simulink library "halin"  (R2021b)
settings: Solver=VariableStepAuto  StartTime=0.0  StopTime=10.0  RelTol=1e-3
undefined symbols (not defined in the file): KHAL_CAN1ABM1E2E_flg, KHAL_CAN1ESC1E2E_flg, KHAL_CAN1ESC5E2E_flg, KHAL_CAN1ESC7E2E_flg, KHAL_CAN1FCM2E2E_flg, KHAL_CAN1FCM3E2E_flg, KHAL_CAN1FCM4E2E_flg, KHAL_CAN3BMS1E2E_flg, KHAL_CAN3BMS6E2E_flg, KHAL_CAN3CCU1E2E_flg, KHAL_CAN3CCU2E2E_flg, KHAL_CAN3MCUF1E2E_flg, KHAL_CAN3MCUR1E2E_flg, KHAL_CAN3Shifter1E2E_flg, TRUE
libraries: simulink x420, FVT_lib x149, hcu_lib x49
(part 12 of 14)

== system halin/HAL_IN/CAN1/ABM1/LifeCountABM1 ==
  LifeCount_ABM1 : Inport
  UnitConverter : DataTypeConversion  OutDataTypeStr=uint8
  VHAL_LifeCountABM1_enum : Outport
  wires:
  UnitConverter/1 -> VHAL_LifeCountABM1_enum/1
  LifeCount_ABM1/1 -> UnitConverter/1

== system halin/HAL_IN/CAN1/ABM1/PsngrSeatBeltCmd ==
  PsngrSeatBeltCmd : Inport
  UnitConverter : DataTypeConversion  OutDataTypeStr=uint8
  VHAL_PsngrSeatBeltCmd_flg : Outport
  wires:
  UnitConverter/1 -> VHAL_PsngrSeatBeltCmd_flg/1
  PsngrSeatBeltCmd/1 -> UnitConverter/1

== system halin/HAL_IN/CAN1/ABM1/RCenterSeatBeltCmd ==
  RCenterSeatBeltCmd : Inport
  UnitConverter : DataTypeConversion  OutDataTypeStr=uint8
  VHAL_RCenterSeatBeltCmd_flg : Outport
  wires:
  UnitConverter/1 -> VHAL_RCenterSeatBeltCmd_flg/1
  RCenterSeatBeltCmd/1 -> UnitConverter/1

== system halin/HAL_IN/CAN1/ABM1/RDriverSeatBeltCmd ==
  RDriverSeatBeltCmd : Inport
  UnitConverter : DataTypeConversion  OutDataTypeStr=uint8
  VHAL_RDriverSeatBeltCmd_flg : Outport
  wires:
  UnitConverter/1 -> VHAL_RDriverSeatBeltCmd_flg/1
  RDriverSeatBeltCmd/1 -> UnitConverter/1

== system halin/HAL_IN/CAN1/ABM1/RPsngrSeatBeltCmd ==
  RPsngrSeatBeltCmd : Inport
  UnitConverter : DataTypeConversion  OutDataTypeStr=uint8
  VHAL_RPsngrSeatBeltCmd_flg : Outport
  wires:
  UnitConverter/1 -> VHAL_RPsngrSeatBeltCmd_flg/1
  RPsngrSeatBeltCmd/1 -> UnitConverter/1

== system halin/HAL_IN/CAN1/EPAS1/DriIntend ==
  DriIntend : Inport
  UnitConverter : DataTypeConversion  OutDataTypeStr=uint8
  VHAL_DriIntend_enum : Outport
  wires:
  UnitConverter/1 -> VHAL_DriIntend_enum/1
  DriIntend/1 -> UnitConverter/1

== system halin/HAL_IN/CAN1/EPAS1/EPSAOIControl ==
  EPS_AOI_Control : Inport
  UnitConverter : DataTypeConversion  OutDataTypeStr=uint8
  VHAL_EPSAOIControl_enum : Outport
  wires:
  UnitConverter/1 -> VHAL_EPSAOIControl_enum/1
  EPS_AOI_Control/1 -> UnitConverter/1

== system halin/HAL_IN/CAN1/EPAS2/SASAngle ==
  SAS_Angle : Inport
  UnitConverter : DataTypeConversion  OutDataTypeStr=uint16
  convert_in : FVT_lib/hal/convert_in  gain=0.1  offset=-900
  VHAL_SASAngle_Deg : Outport
  wires:
  convert_in/1 -> VHAL_SASAngle_Deg/1
  UnitConverter/1 -> convert_in/1
  SAS_Angle/1 -> UnitConverter/1

== system halin/HAL_IN/CAN1/EPAS2/SASCAL ==
  SAS_CAL : Inport
  UnitConverter : DataTypeConversion  OutDataTypeStr=uint8
  VHAL_SASCAL_flg : Outport
  wires:
  UnitConverter/1 -> VHAL_SASCAL_flg/1
  SAS_CAL/1 -> UnitConverter/1

== system halin/HAL_IN/CAN1/EPAS2/SASSpeed ==
  SAS_Speed : Inport
  UnitConverter : DataTypeConversion  OutDataTypeStr=uint8
  convert_in : FVT_lib/hal/convert_in  gain=4  offset=0
  VHAL_SASSpeed_degps : Outport
  wires:
  convert_in/1 -> VHAL_SASSpeed_degps/1
  UnitConverter/1 -> convert_in/1
  SAS_Speed/1 -> UnitConverter/1

== system halin/HAL_IN/CAN1/EPAS2/SASSpeedValid ==
  SAS_Speed_Valid : Inport
  UnitConverter : DataTypeConversion  OutDataTypeStr=uint8
  VHAL_SASSpeedValid_flg : Outport
  wires:
  UnitConverter/1 -> VHAL_SASSpeedValid_flg/1
  SAS_Speed_Valid/1 -> UnitConverter/1

== system halin/HAL_IN/CAN1/EPAS2/SASV ==
  SAS_V : Inport
  UnitConverter : DataTypeConversion  OutDataTypeStr=uint8
  VHAL_SASV_flg : Outport
  wires:
  UnitConverter/1 -> VHAL_SASV_flg/1
  SAS_V/1 -> UnitConverter/1

== system halin/HAL_IN/CAN1/EPB1/DOASta ==
  DOA_Sta : Inport
  UnitConverter : DataTypeConversion  OutDataTypeStr=uint8
  VHAL_DOASta_flg : Outport
  wires:
  UnitConverter/1 -> VHAL_DOASta_flg/1
  DOA_Sta/1 -> UnitConverter/1

== system halin/HAL_IN/CAN1/EPB1/EPBCarWashMode ==
  EPBCarWashMode : Inport
  UnitConverter : DataTypeConversion  OutDataTypeStr=uint8
  VHAL_EPBCarWashMode_flg : Outport
  wires:
  UnitConverter/1 -> VHAL_EPBCarWashMode_flg/1
  EPBCarWashMode/1 -> UnitConverter/1

== system halin/HAL_IN/CAN1/EPB1/EPBErrSta ==
  EPBErrSta : Inport
  UnitConverter : DataTypeConversion  OutDataTypeStr=uint8
  VHAL_EPBErrSta_enum : Outport
  wires:
  UnitConverter/1 -> VHAL_EPBErrSta_enum/1
  EPBErrSta/1 -> UnitConverter/1

== system halin/HAL_IN/CAN1/EPB1/EPBExtApplyAvail ==
  EPBExtApplyAvail : Inport
  UnitConverter : DataTypeConversion  OutDataTypeStr=uint8
  VHAL_EPBExtApplyAvail_flg : Outport
  wires:
  UnitConverter/1 -> VHAL_EPBExtApplyAvail_flg/1
  EPBExtApplyAvail/1 -> UnitConverter/1

== system halin/HAL_IN/CAN1/EPB1/EPBExtReleaseAvail ==
  EPBExtReleaseAvail : Inport
  UnitConverter : DataTypeConversion  OutDataTypeStr=uint8
  VHAL_EPBExtReleaseAvail_flg : Outport
  wires:
  UnitConverter/1 -> VHAL_EPBExtReleaseAvail_flg/1
  EPBExtReleaseAvail/1 -> UnitConverter/1

== system halin/HAL_IN/CAN1/EPB1/EPBSta ==
  EPBSta : Inport
  UnitConverter : DataTypeConversion  OutDataTypeStr=uint8
  VHAL_EPBSta_enum : Outport
  wires:
  UnitConverter/1 -> VHAL_EPBSta_enum/1
  EPBSta/1 -> UnitConverter/1

== system halin/HAL_IN/CAN1/ESC1/ESC1CS ==
  ESC1_CS : Inport
  UnitConverter : DataTypeConversion  OutDataTypeStr=uint8
  VHAL_ESC1CS_enum : Outport
  wires:
  UnitConverter/1 -> VHAL_ESC1CS_enum/1
  ESC1_CS/1 -> UnitConverter/1

== system halin/HAL_IN/CAN1/ESC1/ESC1RC ==
  ESC1_RC : Inport
  UnitConverter : DataTypeConversion  OutDataTypeStr=uint8
  VHAL_ESC1RC_enum : Outport
  wires:
  UnitConverter/1 -> VHAL_ESC1RC_enum/1
  ESC1_RC/1 -> UnitConverter/1

== system halin/HAL_IN/CAN1/ESC1/FrPTCSActive ==
  Fr_PTCS_Active : Inport
  UnitConverter : DataTypeConversion  OutDataTypeStr=uint8
  VHAL_FrPTCSActive_flg : Outport
  wires:
  UnitConverter/1 -> VHAL_FrPTCSActive_flg/1
  Fr_PTCS_Active/1 -> UnitConverter/1

== system halin/HAL_IN/CAN1/ESC1/FrntAxlTrqReqDrv ==
  FrntAxlTrqReq_Drv : Inport
  UnitConverter : DataTypeConversion  OutDataTypeStr=uint16
  convert_in : FVT_lib/hal/convert_in  gain=0.5  offset=-5300
  VHAL_FrntAxlTrqReqDrv_Nm : Outport
  wires:
  convert_in/1 -> VHAL_FrntAxlTrqReqDrv_Nm/1
  UnitConverter/1 -> convert_in/1
  FrntAxlTrqReq_Drv/1 -> UnitConverter/1

== system halin/HAL_IN/CAN1/ESC1/RearAxlTrqReqDrv ==
  RearAxlTrqReq_Drv : Inport
  UnitConverter : DataTypeConversion  OutDataTypeStr=uint16
  convert_in : FVT_lib/hal/convert_in  gain=0.5  offset=-5300
  VHAL_RearAxlTrqReqDrv_Nm : Outport
  wires:
  convert_in/1 -> VHAL_RearAxlTrqReqDrv_Nm/1
  UnitConverter/1 -> convert_in/1
  RearAxlTrqReq_Drv/1 -> UnitConverter/1

== system halin/HAL_IN/CAN1/ESC1/RrPTCSActive ==
  Rr_PTCS_Active : Inport
  UnitConverter : DataTypeConversion  OutDataTypeStr=uint8
  VHAL_RrPTCSActive_flg : Outport
  wires:
  UnitConverter/1 -> VHAL_RrPTCSActive_flg/1
  Rr_PTCS_Active/1 -> UnitConverter/1

== system halin/HAL_IN/CAN1/ESC1/VehSpeed ==
  VehSpeed : Inport
  UnitConverter : DataTypeConversion  OutDataTypeStr=uint16
  convert_in : FVT_lib/hal/convert_in  gain=0.125  offset=0
  VHAL_VehSpeed_kph : Outport
  wires:
  convert_in/1 -> VHAL_VehSpeed_kph/1
  UnitConverter/1 -> convert_in/1
  VehSpeed/1 -> UnitConverter/1

== system halin/HAL_IN/CAN1/ESC2/LFPulseCount ==
  LF_PulseCount : Inport
  UnitConverter : DataTypeConversion  OutDataTypeStr=uint8
  VHAL_LFPulseCount_enum : Outport
  wires:
  UnitConverter/1 -> VHAL_LFPulseCount_enum/1
  LF_PulseCount/1 -> UnitConverter/1

== system halin/HAL_IN/CAN1/ESC2/LFPulseCountV ==
  LF_PulseCount_V : Inport
  UnitConverter : DataTypeConversion  OutDataTypeStr=uint8
  VHAL_LFPulseCountV_flg : Outport
  wires:
  UnitConverter/1 -> VHAL_LFPulseCountV_flg/1
  LF_PulseCount_V/1 -> UnitConverter/1

== system halin/HAL_IN/CAN1/ESC2/LFRawWhlSpeed ==
  LF_RawWhlSpeed : Inport
  UnitConverter : DataTypeConversion  OutDataTypeStr=uint16
  convert_in : FVT_lib/hal/convert_in  gain=0.0625  offset=0
  VHAL_LFRawWhlSpeed_kph : Outport
  wires:
  convert_in/1 -> VHAL_LFRawWhlSpeed_kph/1
  UnitConverter/1 -> convert_in/1
  LF_RawWhlSpeed/1 -> UnitConverter/1

== system halin/HAL_IN/CAN1/ESC2/LFRawWhlSpeedV ==
  LF_RawWhlSpeed_V : Inport
  UnitConverter : DataTypeConversion  OutDataTypeStr=uint8
  VHAL_LFRawWhlSpeedV_flg : Outport
  wires:
  UnitConverter/1 -> VHAL_LFRawWhlSpeedV_flg/1
  LF_RawWhlSpeed_V/1 -> UnitConverter/1

== system halin/HAL_IN/CAN1/ESC2/LFWhlRotDir ==
  LF_WhlRotDir : Inport
  UnitConverter : DataTypeConversion  OutDataTypeStr=uint8
  VHAL_LFWhlRotDir_enum : Outport
  wires:
  UnitConverter/1 -> VHAL_LFWhlRotDir_enum/1
  LF_WhlRotDir/1 -> UnitConverter/1

== system halin/HAL_IN/CAN1/ESC2/RFPulseCount ==
  RF_PulseCount : Inport
  UnitConverter : DataTypeConversion  OutDataTypeStr=uint8
  VHAL_RFPulseCount_enum : Outport
  wires:
  UnitConverter/1 -> VHAL_RFPulseCount_enum/1
  RF_PulseCount/1 -> UnitConverter/1

== system halin/HAL_IN/CAN1/ESC2/RFPulseCountV ==
  RF_PulseCount_V : Inport
  UnitConverter : DataTypeConversion  OutDataTypeStr=uint8
  VHAL_RFPulseCountV_flg : Outport
  wires:
  UnitConverter/1 -> VHAL_RFPulseCountV_flg/1
  RF_PulseCount_V/1 -> UnitConverter/1

== system halin/HAL_IN/CAN1/ESC2/RFRawWhlSpeed ==
  RF_RawWhlSpeed : Inport
  UnitConverter : DataTypeConversion  OutDataTypeStr=uint16
  convert_in : FVT_lib/hal/convert_in  gain=0.0625  offset=0
  VHAL_RFRawWhlSpeed_kph : Outport
  wires:
  convert_in/1 -> VHAL_RFRawWhlSpeed_kph/1
  UnitConverter/1 -> convert_in/1
  RF_RawWhlSpeed/1 -> UnitConverter/1

== system halin/HAL_IN/CAN1/ESC2/RFRawWhlSpeedV ==
  RF_RawWhlSpeed_V : Inport
  UnitConverter : DataTypeConversion  OutDataTypeStr=uint8
  VHAL_RFRawWhlSpeedV_flg : Outport
  wires:
  UnitConverter/1 -> VHAL_RFRawWhlSpeedV_flg/1
  RF_RawWhlSpeed_V/1 -> UnitConverter/1

== system halin/HAL_IN/CAN1/ESC2/RFWhlRotDir ==
  RF_WhlRotDir : Inport
  UnitConverter : DataTypeConversion  OutDataTypeStr=uint8
  VHAL_RFWhlRotDir_enum : Outport
  wires:
  UnitConverter/1 -> VHAL_RFWhlRotDir_enum/1
  RF_WhlRotDir/1 -> UnitConverter/1

== system halin/HAL_IN/CAN1/ESC3/LRPulseCount ==
  LR_PulseCount : Inport
  UnitConverter : DataTypeConversion  OutDataTypeStr=uint8
  VHAL_LRPulseCount_enum : Outport
  wires:
  UnitConverter/1 -> VHAL_LRPulseCount_enum/1
  LR_PulseCount/1 -> UnitConverter/1

== system halin/HAL_IN/CAN1/ESC3/LRPulseCountV ==
  LR_PulseCount_V : Inport
  UnitConverter : DataTypeConversion  OutDataTypeStr=uint8
  VHAL_LRPulseCountV_flg : Outport
  wires:
  UnitConverter/1 -> VHAL_LRPulseCountV_flg/1
  LR_PulseCount_V/1 -> UnitConverter/1

== system halin/HAL_IN/CAN1/ESC3/LRRawWhlSpeed ==
  LR_RawWhlSpeed : Inport
  UnitConverter : DataTypeConversion  OutDataTypeStr=uint16
  convert_in : FVT_lib/hal/convert_in  gain=0.0625  offset=0
  VHAL_LRRawWhlSpeed_kph : Outport
  wires:
  convert_in/1 -> VHAL_LRRawWhlSpeed_kph/1
  UnitConverter/1 -> convert_in/1
  LR_RawWhlSpeed/1 -> UnitConverter/1

== system halin/HAL_IN/CAN1/ESC3/LRRawWhlSpeedV ==
  LR_RawWhlSpeed_V : Inport
  UnitConverter : DataTypeConversion  OutDataTypeStr=uint8
  VHAL_LRRawWhlSpeedV_flg : Outport
  wires:
  UnitConverter/1 -> VHAL_LRRawWhlSpeedV_flg/1
  LR_RawWhlSpeed_V/1 -> UnitConverter/1

== system halin/HAL_IN/CAN1/ESC3/LRWhlRotDir ==
  LR_WhlRotDir : Inport
  UnitConverter : DataTypeConversion  OutDataTypeStr=uint8
  VHAL_LRWhlRotDir_enum : Outport
  wires:
  UnitConverter/1 -> VHAL_LRWhlRotDir_enum/1
  LR_WhlRotDir/1 -> UnitConverter/1

== system halin/HAL_IN/CAN1/ESC3/RRPulseCount ==
  RR_PulseCount : Inport
  UnitConverter : DataTypeConversion  OutDataTypeStr=uint8
  VHAL_RRPulseCount_enum : Outport
  wires:
  UnitConverter/1 -> VHAL_RRPulseCount_enum/1
  RR_PulseCount/1 -> UnitConverter/1

== system halin/HAL_IN/CAN1/ESC3/RRPulseCountV ==
  RR_PulseCount_V : Inport
  UnitConverter : DataTypeConversion  OutDataTypeStr=uint8
  VHAL_RRPulseCountV_flg : Outport
  wires:
  UnitConverter/1 -> VHAL_RRPulseCountV_flg/1
  RR_PulseCount_V/1 -> UnitConverter/1

== system halin/HAL_IN/CAN1/ESC3/RRRawWhlSpeed ==
  RR_RawWhlSpeed : Inport
  UnitConverter : DataTypeConversion  OutDataTypeStr=uint16
  convert_in : FVT_lib/hal/convert_in  gain=0.0625  offset=0
  VHAL_RRRawWhlSpeed_kph : Outport
  wires:
  convert_in/1 -> VHAL_RRRawWhlSpeed_kph/1
  UnitConverter/1 -> convert_in/1
  RR_RawWhlSpeed/1 -> UnitConverter/1

== system halin/HAL_IN/CAN1/ESC3/RRRawWhlSpeedV ==
  RR_RawWhlSpeed_V : Inport
  UnitConverter : DataTypeConversion  OutDataTypeStr=uint8
  VHAL_RRRawWhlSpeedV_flg : Outport
  wires:
  UnitConverter/1 -> VHAL_RRRawWhlSpeedV_flg/1
  RR_RawWhlSpeed_V/1 -> UnitConverter/1

== system halin/HAL_IN/CAN1/ESC3/RRWhlRotDir ==
  RR_WhlRotDir : Inport
  UnitConverter : DataTypeConversion  OutDataTypeStr=uint8
  VHAL_RRWhlRotDir_enum : Outport
  wires:
  UnitConverter/1 -> VHAL_RRWhlRotDir_enum/1
  RR_WhlRotDir/1 -> UnitConverter/1

== system halin/HAL_IN/CAN1/ESC4/ABSActive ==
  ABS_Active : Inport
  UnitConverter : DataTypeConversion  OutDataTypeStr=uint8
  VHAL_ABSActive_flg : Outport
  wires:
  UnitConverter/1 -> VHAL_ABSActive_flg/1
  ABS_Active/1 -> UnitConverter/1

== system halin/HAL_IN/CAN1/ESC4/ABSFailed ==
  ABS_Failed : Inport
  UnitConverter : DataTypeConversion  OutDataTypeStr=uint8
  VHAL_ABSFailed_flg : Outport
  wires:
  UnitConverter/1 -> VHAL_ABSFailed_flg/1
  ABS_Failed/1 -> UnitConverter/1

== system halin/HAL_IN/CAN1/ESC4/AVHActive ==
  AVH_Active : Inport
  UnitConverter : DataTypeConversion  OutDataTypeStr=uint8
  VHAL_AVHActive_flg : Outport
  wires:
  UnitConverter/1 -> VHAL_AVHActive_flg/1
  AVH_Active/1 -> UnitConverter/1

== system halin/HAL_IN/CAN1/ESC4/AVHFailed ==
  AVH_Failed : Inport
  UnitConverter : DataTypeConversion  OutDataTypeStr=uint8
  VHAL_AVHFailed_flg : Outport
  wires:
  UnitConverter/1 -> VHAL_AVHFailed_flg/1
  AVH_Failed/1 -> UnitConverter/1

== system halin/HAL_IN/CAN1/ESC4/BTCSActive ==
  BTCS_Active : Inport
  UnitConverter : DataTypeConversion  OutDataTypeStr=uint8
  VHAL_BTCSActive_flg : Outport
  wires:
  UnitConverter/1 -> VHAL_BTCSActive_flg/1
  BTCS_Active/1 -> UnitConverter/1

== system halin/HAL_IN/CAN1/ESC4/EBDActive ==
  EBD_Active : Inport
  UnitConverter : DataTypeConversion  OutDataTypeStr=uint8
  VHAL_EBDActive_flg : Outport
  wires:
  UnitConverter/1 -> VHAL_EBDActive_flg/1
  EBD_Active/1 -> UnitConverter/1

== system halin/HAL_IN/CAN1/ESC4/EBDFailed ==
  EBD_Failed : Inport
  UnitConverter : DataTypeConversion  OutDataTypeStr=uint8
  VHAL_EBDFailed_flg : Outport
  wires:
  UnitConverter/1 -> VHAL_EBDFailed_flg/1
  EBD_Failed/1 -> UnitConverter/1

== system halin/HAL_IN/CAN1/ESC4/ESCActive ==
  ESC_Active : Inport
  UnitConverter : DataTypeConversion  OutDataTypeStr=uint8
  VHAL_ESCActive_flg : Outport
  wires:
  UnitConverter/1 -> VHAL_ESCActive_flg/1
  ESC_Active/1 -> UnitConverter/1

== system halin/HAL_IN/CAN1/ESC4/ESCFailed ==
  ESC_Failed : Inport
  UnitConverter : DataTypeConversion  OutDataTypeStr=uint8
  VHAL_ESCFailed_flg : Outport
  wires:
  UnitConverter/1 -> VHAL_ESCFailed_flg/1
  ESC_Failed/1 -> UnitConverter/1

== system halin/HAL_IN/CAN1/ESC4/ESSActive ==
  ESS_Active : Inport
  UnitConverter : DataTypeConversion  OutDataTypeStr=uint8
  VHAL_ESSActive_flg : Outport
  wires:
  UnitConverter/1 -> VHAL_ESSActive_flg/1
  ESS_Active/1 -> UnitConverter/1

== system halin/HAL_IN/CAN1/ESC4/GRADE ==
  GRADE : Inport
  UnitConverter : DataTypeConversion  OutDataTypeStr=uint8
  convert_in : FVT_lib/hal/convert_in  gain=0.35433  offset=-45
  VHAL_GRADE_Deg : Outport
  wires:
  convert_in/1 -> VHAL_GRADE_Deg/1
  UnitConverter/1 -> convert_in/1
  GRADE/1 -> UnitConverter/1

== system halin/HAL_IN/CAN1/ESC4/HBBActive ==
  HBB_Active : Inport
  UnitConverter : DataTypeConversion  OutDataTypeStr=uint8
  VHAL_HBBActive_flg : Outport
  wires:
  UnitConverter/1 -> VHAL_HBBActive_flg/1
  HBB_Active/1 -> UnitConverter/1

== system halin/HAL_IN/CAN1/ESC4/HBBFailed ==
  HBB_Failed : Inport
  UnitConverter : DataTypeConversion  OutDataTypeStr=uint8
  VHAL_HBBFailed_flg : Outport
  wires:
  UnitConverter/1 -> VHAL_HBBFailed_flg/1
  HBB_Failed/1 -> UnitConverter/1

== system halin/HAL_IN/CAN1/ESC4/HDDActive ==
  HDD_Active : Inport
  UnitConverter : DataTypeConversion  OutDataTypeStr=uint8
  VHAL_HDDActive_flg : Outport
  wires:
  UnitConverter/1 -> VHAL_HDDActive_flg/1
  HDD_Active/1 -> UnitConverter/1

== system halin/HAL_IN/CAN1/ESC4/HDDFailed ==
  HDD_Failed : Inport
  UnitConverter : DataTypeConversion  OutDataTypeStr=uint8
  VHAL_HDDFailed_flg : Outport
  wires:
  UnitConverter/1 -> VHAL_HDDFailed_flg/1
  HDD_Failed/1 -> UnitConverter/1

== system halin/HAL_IN/CAN1/ESC4/HSAActive ==
  HSA_Active : Inport
  UnitConverter : DataTypeConversion  OutDataTypeStr=uint8
  VHAL_HSAActive_flg : Outport
  wires:
  UnitConverter/1 -> VHAL_HSAActive_flg/1
  HSA_Active/1 -> UnitConverter/1

== system halin/HAL_IN/CAN1/ESC4/HSAFailed ==
  HSA_Failed : Inport
  UnitConverter : DataTypeConversion  OutDataTypeStr=uint8
  VHAL_HSAFailed_flg : Outport
  wires:
  UnitConverter/1 -> VHAL_HSAFailed_flg/1
  HSA_Failed/1 -> UnitConverter/1

== system halin/HAL_IN/CAN1/ESC4/PBAFailed ==
  PBA_Failed : Inport
  UnitConverter : DataTypeConversion  OutDataTypeStr=uint8
  VHAL_PBAFailed_flg : Outport
  wires:
  UnitConverter/1 -> VHAL_PBAFailed_flg/1
  PBA_Failed/1 -> UnitConverter/1

== system halin/HAL_IN/CAN1/ESC4/TCSActive ==
  TCS_Active : Inport
  UnitConverter : DataTypeConversion  OutDataTypeStr=uint8
  VHAL_TCSActive_flg : Outport
  wires:
  UnitConverter/1 -> VHAL_TCSActive_flg/1
  TCS_Active/1 -> UnitConverter/1

== system halin/HAL_IN/CAN1/ESC4/TCSFailed ==
  TCS_Failed : Inport
  UnitConverter : DataTypeConversion  OutDataTypeStr=uint8
  VHAL_TCSFailed_flg : Outport
  wires:
  UnitConverter/1 -> VHAL_TCSFailed_flg/1
  TCS_Failed/1 -> UnitConverter/1

== system halin/HAL_IN/CAN1/ESC5/BrkSwSta ==
  BrkSw_Sta : Inport
  UnitConverter : DataTypeConversion  OutDataTypeStr=uint8
  VHAL_BrkSwSta_flg : Outport
  wires:
  UnitConverter/1 -> VHAL_BrkSwSta_flg/1
  BrkSw_Sta/1 -> UnitConverter/1

== system halin/HAL_IN/CAN1/ESC5/BrkSwV ==
  BrkSw_V : Inport
  UnitConverter : DataTypeConversion  OutDataTypeStr=uint8
  VHAL_BrkSwV_flg : Outport
  wires:
  UnitConverter/1 -> VHAL_BrkSwV_flg/1
  BrkSw_V/1 -> UnitConverter/1

== system halin/HAL_IN/CAN1/ESC5/ESC5CRC8 ==
  ESC5_CRC8 : Inport
  UnitConverter : DataTypeConversion  OutDataTypeStr=uint8
  VHAL_ESC5CRC8_enum : Outport
  wires:
  UnitConverter/1 -> VHAL_ESC5CRC8_enum/1
  ESC5_CRC8/1 -> UnitConverter/1

== system halin/HAL_IN/CAN1/ESC5/ESC5RC ==
  ESC5_RC : Inport
  UnitConverter : DataTypeConversion  OutDataTypeStr=uint8
  VHAL_ESC5RC_enum : Outport
  wires:
  UnitConverter/1 -> VHAL_ESC5RC_enum/1
  ESC5_RC/1 -> UnitConverter/1

== system halin/HAL_IN/CAN1/ESC5/LatAccel ==
  LatAccel : Inport
  UnitConverter : DataTypeConversion  OutDataTypeStr=uint8
  convert_in : FVT_lib/hal/convert_in  gain=0.01  offset=-1.27
  VHAL_LatAccel_Gps : Outport
  wires:
  convert_in/1 -> VHAL_LatAccel_Gps/1
  UnitConverter/1 -> convert_in/1
  LatAccel/1 -> UnitConverter/1

== system halin/HAL_IN/CAN1/ESC5/LatAccelV ==
  LatAccel_V : Inport
  UnitConverter : DataTypeConversion  OutDataTypeStr=uint8
  VHAL_LatAccelV_flg : Outport
  wires:
  UnitConverter/1 -> VHAL_LatAccelV_flg/1
  LatAccel_V/1 -> UnitConverter/1

== system halin/HAL_IN/CAN1/ESC5/LongAccel ==
  LongAccel : Inport
  UnitConverter : DataTypeConversion  OutDataTypeStr=uint8
  convert_in : FVT_lib/hal/convert_in  gain=0.01  offset=-1.27
  VHAL_LongAccel_Gps : Outport
  wires:
  convert_in/1 -> VHAL_LongAccel_Gps/1
  UnitConverter/1 -> convert_in/1
  LongAccel/1 -> UnitConverter/1

== system halin/HAL_IN/CAN1/ESC5/LongAccelV ==
  LongAccel_V : Inport
  UnitConverter : DataTypeConversion  OutDataTypeStr=uint8
  VHAL_LongAccelV_flg : Outport
  wires:
  UnitConverter/1 -> VHAL_LongAccelV_flg/1
  LongAccel_V/1 -> UnitConverter/1

== system halin/HAL_IN/CAN1/ESC5/MCPressure ==
  MCPressure : Inport
  UnitConverter : DataTypeConversion  OutDataTypeStr=uint16
  convert_in : FVT_lib/hal/convert_in  gain=0.1  offset=-9.7
  VHAL_MCPressure_bar : Outport
  wires:
  convert_in/1 -> VHAL_MCPressure_bar/1
  UnitConverter/1 -> convert_in/1
  MCPressure/1 -> UnitConverter/1

== system halin/HAL_IN/CAN1/ESC5/MCPressureV ==
  MCPressure_V : Inport
  UnitConverter : DataTypeConversion  OutDataTypeStr=uint8
  VHAL_MCPressureV_flg : Outport
  wires:
  UnitConverter/1 -> VHAL_MCPressureV_flg/1
  MCPressure_V/1 -> UnitConverter/1

== system halin/HAL_IN/CAN1/ESC5/YawRate ==
  YawRate : Inport
  UnitConverter : DataTypeConversion  OutDataTypeStr=uint16
  convert_in : FVT_lib/hal/convert_in  gain=0.1  offset=-100
  VHAL_YawRate_degps : Outport
  wires:
  convert_in/1 -> VHAL_YawRate_degps/1
  UnitConverter/1 -> convert_in/1
  YawRate/1 -> UnitConverter/1

== system halin/HAL_IN/CAN1/ESC5/YawRateV ==
  YawRate_V : Inport
  UnitConverter : DataTypeConversion  OutDataTypeStr=uint8
  VHAL_YawRateV_flg : Outport
  wires:
  UnitConverter/1 -> VHAL_YawRateV_flg/1
  YawRate_V/1 -> UnitConverter/1

== system halin/HAL_IN/CAN1/ESC6/ActBrkLampSta ==
  ActBrkLamp_Sta : Inport
  UnitConverter : DataTypeConversion  OutDataTypeStr=uint8
  VHAL_ActBrkLampSta_flg : Outport
  wires:
  UnitConverter/1 -> VHAL_ActBrkLampSta_flg/1
  ActBrkLamp_Sta/1 -> UnitConverter/1

== system halin/HAL_IN/CAN1/ESC6/ESCADASSta ==
  ESC_ADAS_Sta : Inport
  UnitConverter : DataTypeConversion  OutDataTypeStr=uint8
  VHAL_ESCADASSta_enum : Outport
  wires:
  UnitConverter/1 -> VHAL_ESCADASSta_enum/1
  ESC_ADAS_Sta/1 -> UnitConverter/1

== system halin/HAL_IN/CAN1/ESC6/ESCAPSSta ==
  ESC_APS_Sta : Inport
  UnitConverter : DataTypeConversion  OutDataTypeStr=uint8
  VHAL_ESCAPSSta_enum : Outport
  wires:
  UnitConverter/1 -> VHAL_ESCAPSSta_enum/1
  ESC_APS_Sta/1 -> UnitConverter/1

== system halin/HAL_IN/CAN1/ESC6/ESCStandstill ==
  ESC_Standstill : Inport
  UnitConverter : DataTypeConversion  OutDataTypeStr=uint8
  VHAL_ESCStandstill_flg : Outport
  wires:
  UnitConverter/1 -> VHAL_ESCStandstill_flg/1
  ESC_Standstill/1 -> UnitConverter/1

== system halin/HAL_IN/CAN1/ESC7/BrkPedalPos ==
  BrkPedalPos : Inport
  UnitConverter : DataTypeConversion  OutDataTypeStr=uint8
  convert_in : FVT_lib/hal/convert_in  gain=0.4  offset=0
  VHAL_BrkPedalPos_pct : Outport
  wires:
  convert_in/1 -> VHAL_BrkPedalPos_pct/1
  UnitConverter/1 -> convert_in/1
  BrkPedalPos/1 -> UnitConverter/1

== system halin/HAL_IN/CAN1/ESC7/BrkPedalPosSta ==
  BrkPedalPos_Sta : Inport
  UnitConverter : DataTypeConversion  OutDataTypeStr=uint8
  VHAL_BrkPedalPosSta_flg : Outport
  wires:
  UnitConverter/1 -> VHAL_BrkPedalPosSta_flg/1
  BrkPedalPos_Sta/1 -> UnitConverter/1

== system halin/HAL_IN/CAN1/ESC7/ESC7CS ==
  ESC7_CS : Inport
  UnitConverter : DataTypeConversion  OutDataTypeStr=uint8
  VHAL_ESC7CS_enum : Outport
  wires:
  UnitConverter/1 -> VHAL_ESC7CS_enum/1
  ESC7_CS/1 -> UnitConverter/1

== system halin/HAL_IN/CAN1/ESC7/ESC7RC ==
  ESC7_RC : Inport
  UnitConverter : DataTypeConversion  OutDataTypeStr=uint8
  VHAL_ESC7RC_enum : Outport
  wires:
  UnitConverter/1 -> VHAL_ESC7RC_enum/1
  ESC7_RC/1 -> UnitConverter/1

== system halin/HAL_IN/CAN1/ESC7/FrRBCActive ==
  Fr_RBC_Active : Inport
  UnitConverter : DataTypeConversion  OutDataTypeStr=uint8
  VHAL_FrRBCActive_flg : Outport
  wires:
  UnitConverter/1 -> VHAL_FrRBCActive_flg/1
  Fr_RBC_Active/1 -> UnitConverter/1

== system halin/HAL_IN/CAN1/ESC7/FrntAxlTrqReqBrk ==
  FrntAxlTrqReq_Brk : Inport
  UnitConverter : DataTypeConversion  OutDataTypeStr=uint16
  convert_in : FVT_lib/hal/convert_in  gain=0.5  offset=-5300
  VHAL_FrntAxlTrqReqBrk_Nm : Outport
  wires:
  convert_in/1 -> VHAL_FrntAxlTrqReqBrk_Nm/1
  UnitConverter/1 -> convert_in/1
  FrntAxlTrqReq_Brk/1 -> UnitConverter/1

== system halin/HAL_IN/CAN1/ESC7/RDCActive ==
  RDC_Active : Inport
  UnitConverter : DataTypeConversion  OutDataTypeStr=uint8
  VHAL_RDCActive_enum : Outport
  wires:
  UnitConverter/1 -> VHAL_RDCActive_enum/1
  RDC_Active/1 -> UnitConverter/1

== system halin/HAL_IN/CAN1/ESC7/RearAxlTrqReqBrk ==
  RearAxlTrqReq_Brk : Inport
  UnitConverter : DataTypeConversion  OutDataTypeStr=uint16
  convert_in : FVT_lib/hal/convert_in  gain=0.5  offset=-5300
  VHAL_RearAxlTrqReqBrk_Nm : Outport
  wires:
  convert_in/1 -> VHAL_RearAxlTrqReqBrk_Nm/1
  UnitConverter/1 -> convert_in/1
  RearAxlTrqReq_Brk/1 -> UnitConverter/1

== system halin/HAL_IN/CAN1/ESC7/RrRBCActive ==
  Rr_RBC_Active : Inport
  UnitConverter : DataTypeConversion  OutDataTypeStr=uint8
  VHAL_RrRBCActive_flg : Outport
  wires:
  UnitConverter/1 -> VHAL_RrRBCActive_flg/1
  Rr_RBC_Active/1 -> UnitConverter/1

== system halin/HAL_IN/CAN1/FCM2/ACCRequiredAccel ==
  ACC_RequiredAccel : Inport
  UnitConverter : DataTypeConversion  OutDataTypeStr=uint16
  convert_in : FVT_lib/hal/convert_in  gain=0.05  offset=-15
  VHAL_ACCRequiredAccel_mps2 : Outport
  wires:
  convert_in/1 -> VHAL_ACCRequiredAccel_mps2/1
  UnitConverter/1 -> convert_in/1
  ACC_RequiredAccel/1 -> UnitConverter/1

== system halin/HAL_IN/CAN1/FCM2/ACCVehHoldReq ==
  ACC_VehHoldReq : Inport
  UnitConverter : DataTypeConversion  OutDataTypeStr=uint8
  VHAL_ACCVehHoldReq_flg : Outport
  wires:
  UnitConverter/1 -> VHAL_ACCVehHoldReq_flg/1
  ACC_VehHoldReq/1 -> UnitConverter/1

== system halin/HAL_IN/CAN1/FCM2/FCM2Checksum ==
  FCM2_Checksum : Inport
  UnitConverter : DataTypeConversion  OutDataTypeStr=uint8
  VHAL_FCM2Checksum_enum : Outport
  wires:
  UnitConverter/1 -> VHAL_FCM2Checksum_enum/1
  FCM2_Checksum/1 -> UnitConverter/1

== system halin/HAL_IN/CAN1/FCM2/FCM2LifeCount ==
  FCM2_LifeCount : Inport
  UnitConverter : DataTypeConversion  OutDataTypeStr=uint8
  VHAL_FCM2LifeCount_enum : Outport
  wires:
  UnitConverter/1 -> VHAL_FCM2LifeCount_enum/1
  FCM2_LifeCount/1 -> UnitConverter/1

== system halin/HAL_IN/CAN1/FCM3/ACCObjDist ==
  ACC_ObjDist : Inport
  UnitConverter : DataTypeConversion  OutDataTypeStr=uint16
  convert_in : FVT_lib/hal/convert_in  gain=0.1  offset=0
  VHAL_ACCObjDist_m : Outport
  wires:
  convert_in/1 -> VHAL_ACCObjDist_m/1
  UnitConverter/1 -> convert_in/1
  ACC_ObjDist/1 -> UnitConverter/1

== system halin/HAL_IN/CAN1/FCM3/ACCObjRelSpd ==
  ACC_ObjRelSpd : Inport
  UnitConverter : DataTypeConversion  OutDataTypeStr=uint16
  convert_in : FVT_lib/hal/convert_in  gain=0.1  offset=-100
  VHAL_ACCObjRelSpd_mps : Outport
  wires:
  convert_in/1 -> VHAL_ACCObjRelSpd_mps/1
  UnitConverter/1 -> convert_in/1
  ACC_ObjRelSpd/1 -> UnitConverter/1

== system halin/HAL_IN/CAN1/FCM3/ADASForceIdle ==
  ADAS_ForceIdle : Inport
  UnitConverter : DataTypeConversion  OutDataTypeStr=uint8
  VHAL_ADASForceIdle_flg : Outport
  wires:
  UnitConverter/1 -> VHAL_ADASForceIdle_flg/1
  ADAS_ForceIdle/1 -> UnitConverter/1

== system halin/HAL_IN/CAN1/FCM3/FCM3Checksum ==
  FCM3_Checksum : Inport
  UnitConverter : DataTypeConversion  OutDataTypeStr=uint8
  VHAL_FCM3Checksum_enum : Outport
  wires:
  UnitConverter/1 -> VHAL_FCM3Checksum_enum/1
  FCM3_Checksum/1 -> UnitConverter/1

== system halin/HAL_IN/CAN1/FCM3/FCM3LifeCount ==
  FCM3_LifeCount : Inport
  UnitConverter : DataTypeConversion  OutDataTypeStr=uint8
  VHAL_FCM3LifeCount_enum : Outport
  wires:
  UnitConverter/1 -> VHAL_FCM3LifeCount_enum/1
  FCM3_LifeCount/1 -> UnitConverter/1

== system halin/HAL_IN/CAN1/FCM4/ACCSetSpeed ==
  ACCSetSpeed : Inport
  UnitConverter : DataTypeConversion  OutDataTypeStr=uint8
  VHAL_ACCSetSpeed_enum : Outport
  wires:
  UnitConverter/1 -> VHAL_ACCSetSpeed_enum/1
  ACCSetSpeed/1 -> UnitConverter/1

== system halin/HAL_IN/CAN1/FCM4/ACCSetSpeedDisp ==
  ACCSetSpeed_Disp : Inport
  UnitConverter : DataTypeConversion  OutDataTypeStr=uint8
  VHAL_ACCSetSpeedDisp_enum : Outport
  wires:
  UnitConverter/1 -> VHAL_ACCSetSpeedDisp_enum/1
  ACCSetSpeed_Disp/1 -> UnitConverter/1

== system halin/HAL_IN/CAN1/FCM4/ADASACCSta ==
  ADAS_ACC_Sta : Inport
  UnitConverter : DataTypeConversion  OutDataTypeStr=uint8
  VHAL_ADASACCSta_enum : Outport
  wires:
  UnitConverter/1 -> VHAL_ADASACCSta_enum/1
  ADAS_ACC_Sta/1 -> UnitConverter/1

== system halin/HAL_IN/CAN1/FCM4/FCM4Checksum ==
  FCM4_Checksum : Inport
  UnitConverter : DataTypeConversion  OutDataTypeStr=uint8
  VHAL_FCM4Checksum_enum : Outport
  wires:
  UnitConverter/1 -> VHAL_FCM4Checksum_enum/1
  FCM4_Checksum/1 -> UnitConverter/1

== system halin/HAL_IN/CAN1/FCM4/ForceLowBeam ==
  ForceLowBeam : Inport
  UnitConverter : DataTypeConversion  OutDataTypeStr=uint8
  VHAL_ForceLowBeam_enum : Outport
  wires:
  UnitConverter/1 -> VHAL_ForceLowBeam_enum/1
  ForceLowBeam/1 -> UnitConverter/1

== system halin/HAL_IN/CAN1/FCM4/HazardWarningReq ==
  HazardWarningReq : Inport
  UnitConverter : DataTypeConversion  OutDataTypeStr=uint8
  VHAL_HazardWarningReq_flg : Outport
  wires:
  UnitConverter/1 -> VHAL_HazardWarningReq_flg/1
  HazardWarningReq/1 -> UnitConverter/1

== system halin/HAL_IN/CAN1/FCM4/LeftTurnLightReq ==
  LeftTurnLightReq : Inport
  UnitConverter : DataTypeConversion  OutDataTypeStr=uint8
  VHAL_LeftTurnLightReq_flg : Outport
  wires:
  UnitConverter/1 -> VHAL_LeftTurnLightReq_flg/1
  LeftTurnLightReq/1 -> UnitConverter/1

== system halin/HAL_IN/CAN1/FCM4/RightTurnLightReq ==
  RightTurnLightReq : Inport
  UnitConverter : DataTypeConversion  OutDataTypeStr=uint8
  VHAL_RightTurnLightReq_flg : Outport
  wires:
  UnitConverter/1 -> VHAL_RightTurnLightReq_flg/1
  RightTurnLightReq/1 -> UnitConverter/1

== system halin/HAL_IN/CAN1/FCM4/TargetType ==
  Target_Type : Inport
  UnitConverter : DataTypeConversion  OutDataTypeStr=uint16
  VHAL_TargetType_enum : Outport
  wires:
  UnitConverter/1 -> VHAL_TargetType_enum/1
  Target_Type/1 -> UnitConverter/1

== system halin/HAL_IN/CAN1/FCM4/TimeGapLevel ==
  TimeGapLevel : Inport
  UnitConverter : DataTypeConversion  OutDataTypeStr=uint8
  VHAL_TimeGapLevel_enum : Outport
  wires:
  UnitConverter/1 -> VHAL_TimeGapLevel_enum/1
  TimeGapLevel/1 -> UnitConverter/1

== system halin/HAL_IN/CAN1/SRR1/SRRBSDWarnL ==
  SRR_BSD_WarnL : Inport
  UnitConverter : DataTypeConversion  OutDataTypeStr=uint8
  VHAL_SRRBSDWarnL_enum : Outport
  wires:
  UnitConverter/1 -> VHAL_SRRBSDWarnL_enum/1
  SRR_BSD_WarnL/1 -> UnitConverter/1

== system halin/HAL_IN/CAN1/SRR1/SRRBSDWarnR ==
  SRR_BSD_WarnR : Inport
  UnitConverter : DataTypeConversion  OutDataTypeStr=uint8
  VHAL_SRRBSDWarnR_enum : Outport
  wires:
  UnitConverter/1 -> VHAL_SRRBSDWarnR_enum/1
  SRR_BSD_WarnR/1 -> UnitConverter/1

== system halin/HAL_IN/CAN1/SRR1/SRRODAWarnL ==
  SRR_ODA_WarnL : Inport
  UnitConverter : DataTypeConversion  OutDataTypeStr=uint8
  VHAL_SRRODAWarnL_enum : Outport
  wires:
  UnitConverter/1 -> VHAL_SRRODAWarnL_enum/1
  SRR_ODA_WarnL/1 -> UnitConverter/1

== system halin/HAL_IN/CAN1/SRR1/SRRODAWarnR ==
  SRR_ODA_WarnR : Inport
  UnitConverter : DataTypeConversion  OutDataTypeStr=uint8
  VHAL_SRRODAWarnR_enum : Outport
  wires:
  UnitConverter/1 -> VHAL_SRRODAWarnR_enum/1
  SRR_ODA_WarnR/1 -> UnitConverter/1

== system halin/HAL_IN/CAN2/IVI1/AmbLightColorSet ==
  AmbLightColorSet : Inport
  UnitConverter : DataTypeConversion  OutDataTypeStr=uint8
  VHAL_AmbLightColorSet_enum : Outport
  wires:
  UnitConverter/1 -> VHAL_AmbLightColorSet_enum/1
  AmbLightColorSet/1 -> UnitConverter/1

== system halin/HAL_IN/CAN2/IVI1/AmbLightUserSet ==
  AmbLightUserSet : Inport
  UnitConverter : DataTypeConversion  OutDataTypeStr=uint8
  VHAL_AmbLightUserSet_enum : Outport
  wires:
  UnitConverter/1 -> VHAL_AmbLightUserSet_enum/1
  AmbLightUserSet/1 -> UnitConverter/1

== system halin/HAL_IN/CAN2/IVI1/BrkAbnGoReadySW ==
  BrkAbn_GoReady_SW : Inport
  UnitConverter : DataTypeConversion  OutDataTypeStr=uint8
  VHAL_BrkAbnGoReadySW_flg : Outport
  wires:
  UnitConverter/1 -> VHAL_BrkAbnGoReadySW_flg/1
  BrkAbn_GoReady_SW/1 -> UnitConverter/1

== system halin/HAL_IN/CAN2/IVI1/DRAmbLightBrightnessSet ==
  DRAmbLightBrightnessSet : Inport
  UnitConverter : DataTypeConversion  OutDataTypeStr=uint8
  VHAL_DRAmbLightBrightnessSet_pct : Outport
  wires:
  UnitConverter/1 -> VHAL_DRAmbLightBrightnessSet_pct/1
  DRAmbLightBrightnessSet/1 -> UnitConverter/1

== system halin/HAL_IN/CAN2/IVI1/FCPFrEvtBtnACMaxReq ==
  FCP_FrEvt_BtnACMaxReq : Inport
  UnitConverter : DataTypeConversion  OutDataTypeStr=uint8
  VHAL_FCPFrEvtBtnACMaxReq_flg : Outport
  wires:
  UnitConverter/1 -> VHAL_FCPFrEvtBtnACMaxReq_flg/1
  FCP_FrEvt_BtnACMaxReq/1 -> UnitConverter/1

== system halin/HAL_IN/CAN2/IVI1/FCPFrEvtBtnACReq ==
  FCP_FrEvt_BtnACReq : Inport
  UnitConverter : DataTypeConversion  OutDataTypeStr=uint8
  VHAL_FCPFrEvtBtnACReq_flg : Outport
  wires:
  UnitConverter/1 -> VHAL_FCPFrEvtBtnACReq_flg/1
  FCP_FrEvt_BtnACReq/1 -> UnitConverter/1

== system halin/HAL_IN/CAN2/IVI1/FCPFrEvtBtnAutoReq ==
  FCP_FrEvt_BtnAutoReq : Inport
  UnitConverter : DataTypeConversion  OutDataTypeStr=uint8
  VHAL_FCPFrEvtBtnAutoReq_flg : Outport
  wires:
  UnitConverter/1 -> VHAL_FCPFrEvtBtnAutoReq_flg/1
  FCP_FrEvt_BtnAutoReq/1 -> UnitConverter/1

== system halin/HAL_IN/CAN2/IVI1/FCPFrEvtBtnSyncReq ==
  FCP_FrEvt_BtnSyncReq : Inport
  UnitConverter : DataTypeConversion  OutDataTypeStr=uint8
  VHAL_FCPFrEvtBtnSyncReq_flg : Outport
  wires:
  UnitConverter/1 -> VHAL_FCPFrEvtBtnSyncReq_flg/1
  FCP_FrEvt_BtnSyncReq/1 -> UnitConverter/1

== system halin/HAL_IN/CAN2/IVI1/FCPMidEvtBtnAutoReq ==
  FCP_MidEvt_BtnAutoReq : Inport
  UnitConverter : DataTypeConversion  OutDataTypeStr=uint8
  VHAL_FCPMidEvtBtnAutoReq_flg : Outport
  wires:
  UnitConverter/1 -> VHAL_FCPMidEvtBtnAutoReq_flg/1
  FCP_MidEvt_BtnAutoReq/1 -> UnitConverter/1

== system halin/HAL_IN/CAN2/IVI1/IPAmbLightBrightnessSet ==
  IPAmbLightBrightnessSet : Inport
  UnitConverter : DataTypeConversion  OutDataTypeStr=uint8
  VHAL_IPAmbLightBrightnessSet_pct : Outport
  wires:
  UnitConverter/1 -> VHAL_IPAmbLightBrightnessSet_pct/1
  IPAmbLightBrightnessSet/1 -> UnitConverter/1

== system halin/HAL_IN/CAN2/IVI1/IVILockSoundSWSta ==
  IVI_Lock_SoundSW_Sta : Inport
  UnitConverter : DataTypeConversion  OutDataTypeStr=uint8
  VHAL_IVILockSoundSWSta_flg : Outport
  wires:
  UnitConverter/1 -> VHAL_IVILockSoundSWSta_flg/1
  IVI_Lock_SoundSW_Sta/1 -> UnitConverter/1

== system halin/HAL_IN/CAN2/IVI1/IVIOTAUpdSta ==
  IVI_OTA_Upd_Sta : Inport
  UnitConverter : DataTypeConversion  OutDataTypeStr=uint8
  VHAL_IVIOTAUpdSta_enum : Outport
  wires:
  UnitConverter/1 -> VHAL_IVIOTAUpdSta_enum/1
  IVI_OTA_Upd_Sta/1 -> UnitConverter/1

== system halin/HAL_IN/CAN2/IVI1/LINKtoDrive ==
  LINKtoDrive : Inport
  UnitConverter : DataTypeConversion  OutDataTypeStr=uint8
  VHAL_LINKtoDrive_flg : Outport
  wires:
  UnitConverter/1 -> VHAL_LINKtoDrive_flg/1
  LINKtoDrive/1 -> UnitConverter/1

== system halin/HAL_IN/CAN2/IVI1/OTACancelDLReq ==
  OTA_CancelDL_Req : Inport
  UnitConverter : DataTypeConversion  OutDataTypeStr=uint8
  VHAL_OTACancelDLReq_flg : Outport
  wires:
  UnitConverter/1 -> VHAL_OTACancelDLReq_flg/1
  OTA_CancelDL_Req/1 -> UnitConverter/1

== system halin/HAL_IN/CAN2/IVI1/OTACompNTFYPres ==
  OTA_CompNTFY_Pres : Inport
  UnitConverter : DataTypeConversion  OutDataTypeStr=uint8
  VHAL_OTACompNTFYPres_flg : Outport
  wires:
  UnitConverter/1 -> VHAL_OTACompNTFYPres_flg/1
  OTA_CompNTFY_Pres/1 -> UnitConverter/1

== system halin/HAL_IN/CAN2/IVI1/OTADLReq ==
  OTA_DL_Req : Inport
  UnitConverter : DataTypeConversion  OutDataTypeStr=uint8
  VHAL_OTADLReq_flg : Outport
  wires:
  UnitConverter/1 -> VHAL_OTADLReq_flg/1
  OTA_DL_Req/1 -> UnitConverter/1

== system halin/HAL_IN/CAN2/IVI1/OTASuspendDLReq ==
  OTA_SuspendDL_Req : Inport
  UnitConverter : DataTypeConversion  OutDataTypeStr=uint8
  VHAL_OTASuspendDLReq_flg : Outport
  wires:
  UnitConverter/1 -> VHAL_OTASuspendDLReq_flg/1
  OTA_SuspendDL_Req/1 -> UnitConverter/1

== system halin/HAL_IN/CAN2/IVI1/OTAUpdStartReq ==
  OTA_UpdStart_Req : Inport
  UnitConverter : DataTypeConversion  OutDataTypeStr=uint8
  VHAL_OTAUpdStartReq_flg : Outport
  wires:
  UnitConverter/1 -> VHAL_OTAUpdStartReq_flg/1
  OTA_UpdStart_Req/1 -> UnitConverter/1

== system halin/HAL_IN/CAN2/IVI1/OpenDrOpenWdoSW ==
  OpenDrOpenWdo_SW : Inport
  UnitConverter : DataTypeConversion  OutDataTypeStr=uint8
  VHAL_OpenDrOpenWdoSW_flg : Outport
  wires:
  UnitConverter/1 -> VHAL_OpenDrOpenWdoSW_flg/1
  OpenDrOpenWdo_SW/1 -> UnitConverter/1

== system halin/HAL_IN/CAN2/IVI1/PWCLOSEIMD ==
  PW_CLOSE_IMD : Inport
  UnitConverter : DataTypeConversion  OutDataTypeStr=uint8
  VHAL_PWCLOSEIMD_flg : Outport
  wires:
  UnitConverter/1 -> VHAL_PWCLOSEIMD_flg/1
  PW_CLOSE_IMD/1 -> UnitConverter/1

== system halin/HAL_IN/CAN2/IVI1/PWCONTINUEUSE ==
  PW_CONTINUE_USE : Inport
  UnitConverter : DataTypeConversion  OutDataTypeStr=uint8
  VHAL_PWCONTINUEUSE_flg : Outport
  wires:
  UnitConverter/1 -> VHAL_PWCONTINUEUSE_flg/1
  PW_CONTINUE_USE/1 -> UnitConverter/1

== system halin/HAL_IN/CAN2/IVI1/SchedOTAwake ==
  Sched_OTA_wake : Inport
  UnitConverter : DataTypeConversion  OutDataTypeStr=uint8
  VHAL_SchedOTAwake_flg : Outport
  wires:
  UnitConverter/1 -> VHAL_SchedOTAwake_flg/1
  Sched_OTA_wake/1 -> UnitConverter/1

== system halin/HAL_IN/CAN2/IVI1/SmartEcoModeSW ==
  SmartEco_Mode_SW : Inport
  UnitConverter : DataTypeConversion  OutDataTypeStr=uint8
  VHAL_SmartEcoModeSW_flg : Outport
  wires:
  UnitConverter/1 -> VHAL_SmartEcoModeSW_flg/1
  SmartEco_Mode_SW/1 -> UnitConverter/1

== system halin/HAL_IN/CAN2/IVI1/UpdCountdownCancel ==
  Upd_Countdown_Cancel : Inport
  UnitConverter : DataTypeConversion  OutDataTypeStr=uint8
  VHAL_UpdCountdownCancel_flg : Outport
  wires:
  UnitConverter/1 -> VHAL_UpdCountdownCancel_flg/1
  Upd_Countdown_Cancel/1 -> UnitConverter/1

== system halin/HAL_IN/CAN2/IVI1/UpdCountdownSkip ==
  Upd_Countdown_Skip : Inport
  UnitConverter : DataTypeConversion  OutDataTypeStr=uint8
  VHAL_UpdCountdownSkip_flg : Outport
  wires:
  UnitConverter/1 -> VHAL_UpdCountdownSkip_flg/1
  Upd_Countdown_Skip/1 -> UnitConverter/1

== system halin/HAL_IN/CAN2/IVI1/VehACModReq ==
  VehACModReq : Inport
  UnitConverter : DataTypeConversion  OutDataTypeStr=uint8
  VHAL_VehACModReq_enum : Outport
  wires:
  UnitConverter/1 -> VHAL_VehACModReq_enum/1
  VehACModReq/1 -> UnitConverter/1

== system halin/HAL_IN/CAN2/IVI2/AVMErrSTA ==
  AVM_Err_STA : Inport
  UnitConverter : DataTypeConversion  OutDataTypeStr=uint8
  VHAL_AVMErrSTA_flg : Outport
  wires:
  UnitConverter/1 -> VHAL_AVMErrSTA_flg/1
  AVM_Err_STA/1 -> UnitConverter/1

== system halin/HAL_IN/CAN2/IVI2/AVMOFFRecButt ==
  AVM_OFF_Rec_Butt : Inport
  UnitConverter : DataTypeConversion  OutDataTypeStr=uint8
  VHAL_AVMOFFRecButt_flg : Outport
  wires:
  UnitConverter/1 -> VHAL_AVMOFFRecButt_flg/1
  AVM_OFF_Rec_Butt/1 -> UnitConverter/1

== system halin/HAL_IN/CAN2/IVI2/AVMParkingmode ==
  AVM_Parking_mode : Inport
  UnitConverter : DataTypeConversion  OutDataTypeStr=uint8
  VHAL_AVMParkingmode_enum : Outport
  wires:
  UnitConverter/1 -> VHAL_AVMParkingmode_enum/1
  AVM_Parking_mode/1 -> UnitConverter/1

== system halin/HAL_IN/CAN2/IVI2/AVMparkingcancel ==
  AVM_parking_cancel : Inport
  UnitConverter : DataTypeConversion  OutDataTypeStr=uint8
  VHAL_AVMparkingcancel_enum : Outport
  wires:
  UnitConverter/1 -> VHAL_AVMparkingcancel_enum/1
  AVM_parking_cancel/1 -> UnitConverter/1

== system halin/HAL_IN/CAN2/IVI2/AVMparkingexcute ==
  AVM_parking_excute : Inport
  UnitConverter : DataTypeConversion  OutDataTypeStr=uint8
  VHAL_AVMparkingexcute_enum : Outport
  wires:
  UnitConverter/1 -> VHAL_AVMparkingexcute_enum/1
  AVM_parking_excute/1 -> UnitConverter/1

== system halin/HAL_IN/CAN2/IVI2/ApproachUnlockSW ==
  Approach_Unlock_SW : Inport
  UnitConverter : DataTypeConversion  OutDataTypeStr=uint8
  VHAL_ApproachUnlockSW_flg : Outport
  wires:
  UnitConverter/1 -> VHAL_ApproachUnlockSW_flg/1
  Approach_Unlock_SW/1 -> UnitConverter/1

== system halin/HAL_IN/CAN2/IVI2/CAASSw ==
  CAAS_Sw : Inport
  UnitConverter : DataTypeConversion  OutDataTypeStr=uint8
  VHAL_CAASSw_enum : Outport
  wires:
  UnitConverter/1 -> VHAL_CAASSw_enum/1
  CAAS_Sw/1 -> UnitConverter/1

== system halin/HAL_IN/CAN2/IVI2/CDLLockButt ==
  CDL_Lock_Butt : Inport
  UnitConverter : DataTypeConversion  OutDataTypeStr=uint8
  VHAL_CDLLockButt_flg : Outport
  wires:
  UnitConverter/1 -> VHAL_CDLLockButt_flg/1
  CDL_Lock_Butt/1 -> UnitConverter/1

== system halin/HAL_IN/CAN2/IVI2/CDLUnlockButt ==
  CDL_Unlock_Butt : Inport
  UnitConverter : DataTypeConversion  OutDataTypeStr=uint8
  VHAL_CDLUnlockButt_flg : Outport
  wires:
  UnitConverter/1 -> VHAL_CDLUnlockButt_flg/1
  CDL_Unlock_Butt/1 -> UnitConverter/1

== system halin/HAL_IN/CAN2/IVI2/DSEATantiset ==
  DSEAT_anti_set : Inport
  UnitConverter : DataTypeConversion  OutDataTypeStr=uint8
  VHAL_DSEATantiset_flg : Outport
  wires:
  UnitConverter/1 -> VHAL_DSEATantiset_flg/1
  DSEAT_anti_set/1 -> UnitConverter/1

== system halin/HAL_IN/CAN2/IVI2/DSEATentryfunset ==
  DSEAT_entryfun_set : Inport
  UnitConverter : DataTypeConversion  OutDataTypeStr=uint8
  VHAL_DSEATentryfunset_flg : Outport
  wires:
  UnitConverter/1 -> VHAL_DSEATentryfunset_flg/1
  DSEAT_entryfun_set/1 -> UnitConverter/1

== system halin/HAL_IN/CAN2/IVI2/DSEATventreq ==
  DSEAT_vent_req : Inport
  UnitConverter : DataTypeConversion  OutDataTypeStr=uint8
  VHAL_DSEATventreq_enum : Outport
  wires:
  UnitConverter/1 -> VHAL_DSEATventreq_enum/1
  DSEAT_vent_req/1 -> UnitConverter/1

== system halin/HAL_IN/CAN2/IVI2/ESCSWCmd ==
  ESC_SW_Cmd : Inport
  UnitConverter : DataTypeConversion  OutDataTypeStr=uint8
  VHAL_ESCSWCmd_enum : Outport
  wires:
  UnitConverter/1 -> VHAL_ESCSWCmd_enum/1
  ESC_SW_Cmd/1 -> UnitConverter/1

== system halin/HAL_IN/CAN2/IVI2/FSOffSw ==
  FS_Off_Sw : Inport
  UnitConverter : DataTypeConversion  OutDataTypeStr=uint8
  VHAL_FSOffSw_enum : Outport
  wires:
  UnitConverter/1 -> VHAL_FSOffSw_enum/1
  FS_Off_Sw/1 -> UnitConverter/1

== system halin/HAL_IN/CAN2/IVI2/FollowMeSW ==
  FollowMeSW : Inport
  UnitConverter : DataTypeConversion  OutDataTypeStr=uint8
  VHAL_FollowMeSW_flg : Outport
  wires:
  UnitConverter/1 -> VHAL_FollowMeSW_flg/1
  FollowMeSW/1 -> UnitConverter/1

== system halin/HAL_IN/CAN2/IVI2/GPSLAT ==
  GPS_LAT : Inport
  UnitConverter : DataTypeConversion  OutDataTypeStr=uint32
  VHAL_GPSLAT_s : Outport
  wires:
  UnitConverter/1 -> VHAL_GPSLAT_s/1
  GPS_LAT/1 -> UnitConverter/1

== system halin/HAL_IN/CAN2/IVI2/GPSLONG ==
  GPS_LONG : Inport
  UnitConverter : DataTypeConversion  OutDataTypeStr=uint32
  VHAL_GPSLONG_enum : Outport
  wires:
  UnitConverter/1 -> VHAL_GPSLONG_enum/1
  GPS_LONG/1 -> UnitConverter/1

== system halin/HAL_IN/CAN2/IVI2/HeadLampSW ==
  HeadLampSW : Inport
  UnitConverter : DataTypeConversion  OutDataTypeStr=uint8
  VHAL_HeadLampSW_enum : Outport
  wires:
  UnitConverter/1 -> VHAL_HeadLampSW_enum/1
  HeadLampSW/1 -> UnitConverter/1

== system halin/HAL_IN/CAN2/IVI2/HoodLatchSW ==
  Hood_Latch_SW : Inport
  UnitConverter : DataTypeConversion  OutDataTypeStr=uint8
  VHAL_HoodLatchSW_enum : Outport
  wires:
  UnitConverter/1 -> VHAL_HoodLatchSW_enum/1
  Hood_Latch_SW/1 -> UnitConverter/1

== system halin/HAL_IN/CAN2/IVI2/IVICreepSWReq ==
  IVI_CreepSW_Req : Inport
  UnitConverter : DataTypeConversion  OutDataTypeStr=uint8
  VHAL_IVICreepSWReq_flg : Outport
  wires:
  UnitConverter/1 -> VHAL_IVICreepSWReq_flg/1
  IVI_CreepSW_Req/1 -> UnitConverter/1

== system halin/HAL_IN/CAN2/IVI2/IVIISAOffsetSpd ==
  IVI_ISA_OffsetSpd : Inport
  UnitConverter : DataTypeConversion  OutDataTypeStr=uint8
  VHAL_IVIISAOffsetSpd_enum : Outport
  wires:
  UnitConverter/1 -> VHAL_IVIISAOffsetSpd_enum/1
  IVI_ISA_OffsetSpd/1 -> UnitConverter/1

== system halin/HAL_IN/CAN2/IVI2/IVINightModeSta ==
  IVI_Night_Mode_Sta : Inport
  UnitConverter : DataTypeConversion  OutDataTypeStr=uint8
  VHAL_IVINightModeSta_flg : Outport
  wires:
  UnitConverter/1 -> VHAL_IVINightModeSta_flg/1
  IVI_Night_Mode_Sta/1 -> UnitConverter/1

== system halin/HAL_IN/CAN2/IVI2/IVIPTGModeSW ==
  IVI_PTG_Mode_SW : Inport
  UnitConverter : DataTypeConversion  OutDataTypeStr=uint8
  VHAL_IVIPTGModeSW_enum : Outport
  wires:
  UnitConverter/1 -> VHAL_IVIPTGModeSW_enum/1
  IVI_PTG_Mode_SW/1 -> UnitConverter/1

== system halin/HAL_IN/CAN2/IVI2/IVIPTGOpenHeight ==
  IVI_PTG_Open_Height : Inport
  UnitConverter : DataTypeConversion  OutDataTypeStr=uint8
  VHAL_IVIPTGOpenHeight_enum : Outport
  wires:
  UnitConverter/1 -> VHAL_IVIPTGOpenHeight_enum/1
  IVI_PTG_Open_Height/1 -> UnitConverter/1

== system halin/HAL_IN/CAN2/IVI2/IVIPTGStaSW ==
  IVI_PTG_Sta_SW : Inport
  UnitConverter : DataTypeConversion  OutDataTypeStr=uint8
  VHAL_IVIPTGStaSW_enum : Outport
  wires:
  UnitConverter/1 -> VHAL_IVIPTGStaSW_enum/1
  IVI_PTG_Sta_SW/1 -> UnitConverter/1

== system halin/HAL_IN/CAN2/IVI2/IVIPTGUSStaSW ==
  IVI_PTG_USSta_SW : Inport
  UnitConverter : DataTypeConversion  OutDataTypeStr=uint8
  VHAL_IVIPTGUSStaSW_flg : Outport
  wires:
  UnitConverter/1 -> VHAL_IVIPTGUSStaSW_flg/1
  IVI_PTG_USSta_SW/1 -> UnitConverter/1

== system halin/HAL_IN/CAN2/IVI2/IVIPWModeReq ==
  IVI_PW_Mode_Req : Inport
  UnitConverter : DataTypeConversion  OutDataTypeStr=uint8
  VHAL_IVIPWModeReq_enum : Outport
  wires:
  UnitConverter/1 -> VHAL_IVIPWModeReq_enum/1
  IVI_PW_Mode_Req/1 -> UnitConverter/1

== system halin/HAL_IN/CAN2/IVI2/IVIPwrLockSW ==
  IVI_PwrLockSW : Inport
  UnitConverter : DataTypeConversion  OutDataTypeStr=uint8
  VHAL_IVIPwrLockSW_enum : Outport
  wires:
  UnitConverter/1 -> VHAL_IVIPwrLockSW_enum/1
  IVI_PwrLockSW/1 -> UnitConverter/1

== system halin/HAL_IN/CAN2/IVI2/IVIPwroffreq ==
  IVI_Pwroff_req : Inport
  UnitConverter : DataTypeConversion  OutDataTypeStr=uint8
  VHAL_IVIPwroffreq_flg : Outport
  wires:
  UnitConverter/1 -> VHAL_IVIPwroffreq_flg/1
  IVI_Pwroff_req/1 -> UnitConverter/1

== system halin/HAL_IN/CAN2/IVI2/IVIRRDefReq ==
  IVI_RR_Def_Req : Inport
  UnitConverter : DataTypeConversion  OutDataTypeStr=uint8
  VHAL_IVIRRDefReq_flg : Outport
  wires:
  UnitConverter/1 -> VHAL_IVIRRDefReq_flg/1
  IVI_RR_Def_Req/1 -> UnitConverter/1

== system halin/HAL_IN/CAN2/IVI2/IVIReqV2L ==
  IVI_Req_V2L : Inport
  UnitConverter : DataTypeConversion  OutDataTypeStr=uint8
  VHAL_IVIReqV2L_flg : Outport
  wires:
  UnitConverter/1 -> VHAL_IVIReqV2L_flg/1
  IVI_Req_V2L/1 -> UnitConverter/1

== system halin/HAL_IN/CAN2/IVI2/IVIScreen ==
  IVI_Screen : Inport
  UnitConverter : DataTypeConversion  OutDataTypeStr=uint8
  VHAL_IVIScreen_enum : Outport
  wires:
  UnitConverter/1 -> VHAL_IVIScreen_enum/1
  IVI_Screen/1 -> UnitConverter/1

== system halin/HAL_IN/CAN2/IVI2/IVIStatus ==
  IVI_Status : Inport
  UnitConverter : DataTypeConversion  OutDataTypeStr=uint8
  VHAL_IVIStatus_flg : Outport
  wires:
  UnitConverter/1 -> VHAL_IVIStatus_flg/1
  IVI_Status/1 -> UnitConverter/1

== system halin/HAL_IN/CAN2/IVI2/IVITriggerreq ==
  IVI_Trigger_req : Inport
  UnitConverter : DataTypeConversion  OutDataTypeStr=uint8
  VHAL_IVITriggerreq_flg : Outport
  wires:
  UnitConverter/1 -> VHAL_IVITriggerreq_flg/1
  IVI_Trigger_req/1 -> UnitConverter/1

== system halin/HAL_IN/CAN2/IVI2/IVIWIMAINSW ==
  IVI_WI_MAIN_SW : Inport
  UnitConverter : DataTypeConversion  OutDataTypeStr=uint8
  VHAL_IVIWIMAINSW_flg : Outport
  wires:
  UnitConverter/1 -> VHAL_IVIWIMAINSW_flg/1
  IVI_WI_MAIN_SW/1 -> UnitConverter/1

== system halin/HAL_IN/CAN2/IVI2/LDrvControlCommand ==
  L_Drv_ControlCommand : Inport
  UnitConverter : DataTypeConversion  OutDataTypeStr=uint8
  VHAL_LDrvControlCommand_pct : Outport
  wires:
  UnitConverter/1 -> VHAL_LDrvControlCommand_pct/1
  L_Drv_ControlCommand/1 -> UnitConverter/1

== system halin/HAL_IN/CAN2/IVI2/LPasControlCommand ==
  L_Pas_ControlCommand : Inport
  UnitConverter : DataTypeConversion  OutDataTypeStr=uint8
  VHAL_LPasControlCommand_pct : Outport
  wires:
  UnitConverter/1 -> VHAL_LPasControlCommand_pct/1
  L_Pas_ControlCommand/1 -> UnitConverter/1

== system halin/HAL_IN/CAN2/IVI2/LRLDControlCommand ==
  L_RLD_ControlCommand : Inport
  UnitConverter : DataTypeConversion  OutDataTypeStr=uint8
  VHAL_LRLDControlCommand_pct : Outport
  wires:
  UnitConverter/1 -> VHAL_LRLDControlCommand_pct/1
  L_RLD_ControlCommand/1 -> UnitConverter/1

== system halin/HAL_IN/CAN2/IVI2/LRRDControlCommand ==
  L_RRD_ControlCommand : Inport
  UnitConverter : DataTypeConversion  OutDataTypeStr=uint8
  VHAL_LRRDControlCommand_pct : Outport
  wires:
  UnitConverter/1 -> VHAL_LRRDControlCommand_pct/1
  L_RRD_ControlCommand/1 -> UnitConverter/1

== system halin/HAL_IN/CAN2/IVI2/MFRDNBrightReq ==
  MFRD_N_Bright_Req : Inport
  UnitConverter : DataTypeConversion  OutDataTypeStr=uint8
  VHAL_MFRDNBrightReq_pct : Outport
  wires:
  UnitConverter/1 -> VHAL_MFRDNBrightReq_pct/1
  MFRD_N_Bright_Req/1 -> UnitConverter/1

== system halin/HAL_IN/CAN2/IVI2/OFFACMODE ==
  OFF_AC_MODE : Inport
  UnitConverter : DataTypeConversion  OutDataTypeStr=uint8
  VHAL_OFFACMODE_enum : Outport
  wires:
  UnitConverter/1 -> VHAL_OFFACMODE_enum/1
  OFF_AC_MODE/1 -> UnitConverter/1

== system halin/HAL_IN/CAN2/IVI2/PSEATventreq ==
  PSEAT_vent_req : Inport
  UnitConverter : DataTypeConversion  OutDataTypeStr=uint8
  VHAL_PSEATventreq_enum : Outport
  wires:
  UnitConverter/1 -> VHAL_PSEATventreq_enum/1
  PSEAT_vent_req/1 -> UnitConverter/1

== system halin/HAL_IN/CAN2/IVI2/PerdV2L ==
  Perd_V2L : Inport
  UnitConverter : DataTypeConversion  OutDataTypeStr=uint8
  VHAL_PerdV2L_enum : Outport
  wires:
  UnitConverter/1 -> VHAL_PerdV2L_enum/1
  Perd_V2L/1 -> UnitConverter/1

== system halin/HAL_IN/CAN2/IVI2/RFogLampSW ==
  RFogLampSW : Inport
  UnitConverter : DataTypeConversion  OutDataTypeStr=uint8
  VHAL_RFogLampSW_flg : Outport
  wires:
  UnitConverter/1 -> VHAL_RFogLampSW_flg/1
  RFogLampSW/1 -> UnitConverter/1
